simulink model "WiperControl"  (R2023b)
settings: Solver=FixedStepAuto  StartTime=0.0  StopTime=20  FixedStep=0.01  RelTol=1e-3
libraries: simulink x1, SignalEditorBlockLib x1
settings Model: LastModifiedBy=Mohamed Majdi
settings OptimizationCC: DefaultParameterBehavior=Inlined  UseDivisionForNetSlopeComputation=on  GainParamInheritBuiltInType=on  UseFloatMulNetSlope=on  OptimizeBlockIOStorage=off  LifeSpan=1  OptimizeDataStoreBuffers=off  BusAssignmentInplaceUpdate=off
settings DebuggingCC: SFUnexpectedBacktrackingDiag=warning  SFNoUnconditionalDefaultTransitionDiag=warning
settings HardwareCC: ProdLongLongMode=on
settings SFSimCC: MATLABDynamicMemAlloc=off
settings RTWCC: GenerateReport=on  BuildConfiguration=Debug  LaunchReport=on
settings CodeAppCC: ForceParamTrailComments=on  MATLABSourceComments=on  EnableCustomComments=on
settings GRTTargetCC: CombineSignalStateStructs=on  SupportVariableSizeSignals=on  MultiInstanceErrorCode=Warning

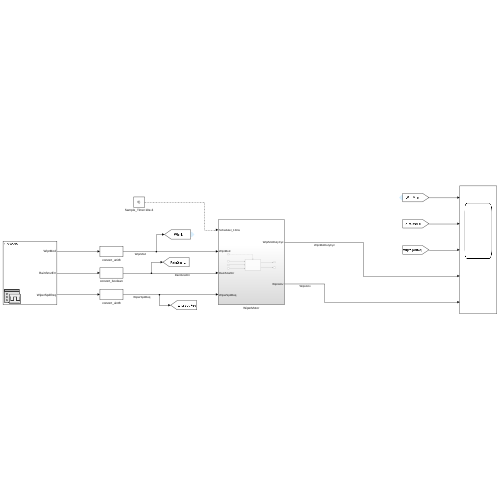
[thumbnail: Simulink's stored preview of the top-level diagram]
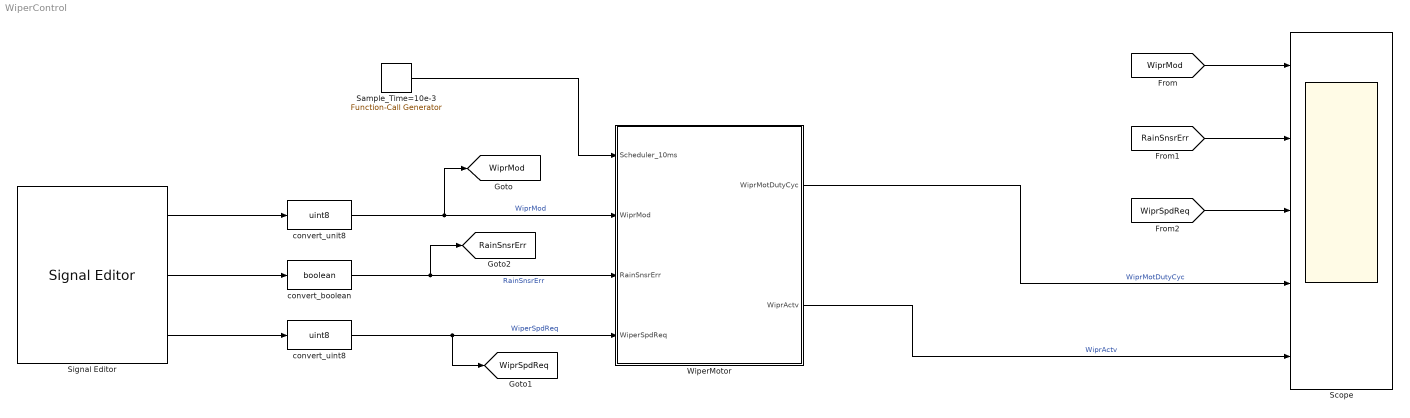
== system WiperControl ==
  Sample_Time=10e-3 : simulink/Ports & Subsystems/Function-Call Generator  sample_time=10e-3  numberOfIterations=1  DisallowWideOutput=off
  Scope : Scope  NumInputPorts=5
  Signal Editor : SignalEditorBlockLib/Signal Editor  FileName=WiperSignals.mat  ActiveScenario=Scenario  ActiveSignal=WiprMod  IsBus=off  OutputBusObjectStr=Bus: BusObject  SampleTime=0  Interpolate=off  ZeroCross=off  OutputAfterFinalValue=Setting to zero  Unit=inherit  PreserveSignalName=on  ApplySigPropsToAllScenarios=on  ApplySigPropsToAllSignals=on
  WiperMotor : Subsystem
  convert_boolean : DataTypeConversion  OutDataTypeStr=boolean  SaturateOnIntegerOverflow=off  RndMeth=Floor
  convert_uint8 : DataTypeConversion  OutDataTypeStr=uint8  SaturateOnIntegerOverflow=off  RndMeth=Floor
  convert_unit8 : DataTypeConversion  OutDataTypeStr=uint8  SaturateOnIntegerOverflow=off  RndMeth=Floor
  tag scope: RainSnsrErr=global, WiprMod=global, WiprSpdReq=global
  wires:
  convert_unit8/1 -> WiperMotor/2(WiprMod), [WiprMod]  "WiprMod"
  Signal Editor/3 -> convert_uint8/1
  Signal Editor/2 -> convert_boolean/1
  Signal Editor/1 -> convert_unit8/1
  [WiprMod] -> Scope/1
  Sample_Time=10e-3/1 -> WiperMotor/1(Scheduler_10ms)
  convert_boolean/1 -> [RainSnsrErr], WiperMotor/3(RainSnsrErr)  "RainSnsrErr"
  convert_uint8/1 -> WiperMotor/4(WiperSpdReq), [WiprSpdReq]  "WiperSpdReq"
  WiperMotor/1(WiprMotDutyCyc) -> Scope/4  "WiprMotDutyCyc"
  WiperMotor/2(WiprActv) -> Scope/5  "WiprActv"
  [RainSnsrErr] -> Scope/2
  [WiprSpdReq] -> Scope/3

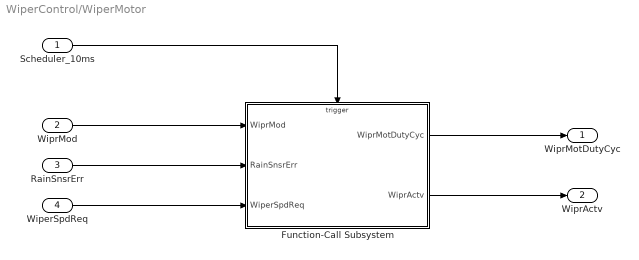
== system WiperControl/WiperMotor ==
  Scheduler_10ms : Inport
  WiprMod : Inport  Port=2  OutDataTypeStr=uint8
  RainSnsrErr : Inport  Port=3  OutDataTypeStr=boolean
  WiperSpdReq : Inport  Port=4  OutDataTypeStr=uint8
  Function-Call Subsystem : Subsystem  TreatAsAtomicUnit=on
  WiprMotDutyCyc : Outport
  WiprActv : Outport  Port=2  OutDataTypeStr=boolean
  wires:
  WiperSpdReq/1 -> Function-Call Subsystem/3(WiperSpdReq)
  Function-Call Subsystem/1(WiprMotDutyCyc) -> WiprMotDutyCyc/1
  Scheduler_10ms/1 -> Function-Call Subsystem/Trigger
  RainSnsrErr/1 -> Function-Call Subsystem/2(RainSnsrErr)
  WiprMod/1 -> Function-Call Subsystem/1(WiprMod)
  Function-Call Subsystem/2(WiprActv) -> WiprActv/1

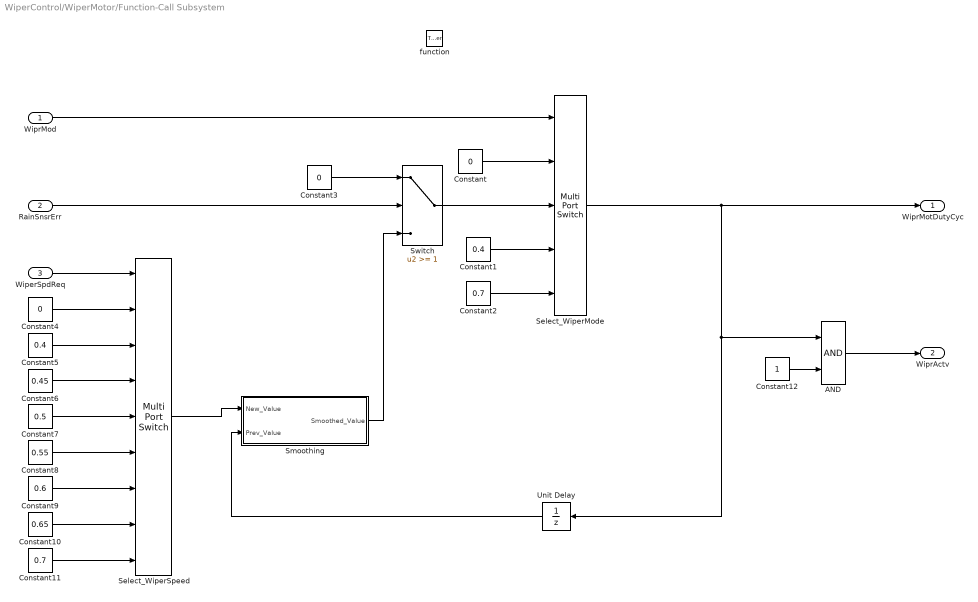
== system WiperControl/WiperMotor/Function-Call Subsystem ==
  WiprMod : Inport
  RainSnsrErr : Inport  Port=2
  WiperSpdReq : Inport  Port=3
  function : TriggerPort  TriggerType=function-call  VariantControl=(inherit)
  AND : Logic  IconShape=distinctive  AllPortsSameDT=off  OutDataTypeStr=boolean
  Constant : Constant  Value=0  OutDataTypeStr=uint8
  Constant1 : Constant  Value=0.4
  Constant10 : Constant  Value=0.65
  Constant11 : Constant  Value=0.7
  Constant12 : Constant
  Constant2 : Constant  Value=0.7
  Constant3 : Constant  Value=0  OutDataTypeStr=uint8
  Constant4 : Constant  Value=0
  Constant5 : Constant  Value=0.4
  Constant6 : Constant  Value=0.45
  Constant7 : Constant  Value=0.5
  Constant8 : Constant  Value=0.55
  Constant9 : Constant  Value=0.6
  Select_WiperMode : MultiPortSwitch  DataPortOrder=Zero-based contiguous  Inputs=4  zeroidx=on  SaturateOnIntegerOverflow=off  InputSameDT=off
  Select_WiperSpeed : MultiPortSwitch  DataPortOrder=Zero-based contiguous  Inputs=8  zeroidx=on  SaturateOnIntegerOverflow=off  InputSameDT=off
  Smoothing : Subsystem  TreatAsAtomicUnit=on
  Switch : Switch  Threshold=1  SaturateOnIntegerOverflow=off  InputSameDT=off
  Unit Delay : UnitDelay  SampleTime=-1  HasFrameUpgradeWarning=on
  WiprMotDutyCyc : Outport  OutDataTypeStr=double
  WiprActv : Outport  Port=2  OutDataTypeStr=boolean
  wires:
  WiprMod/1 -> Select_WiperMode/1
  Select_WiperMode/1 -> WiprMotDutyCyc/1, Unit Delay/1, AND/1
  Constant/1 -> Select_WiperMode/2
  Constant2/1 -> Select_WiperMode/5
  Constant1/1 -> Select_WiperMode/4
  RainSnsrErr/1 -> Switch/2
  Switch/1 -> Select_WiperMode/3
  Constant3/1 -> Switch/1
  WiperSpdReq/1 -> Select_WiperSpeed/1
  Constant4/1 -> Select_WiperSpeed/2
  Constant5/1 -> Select_WiperSpeed/3
  Constant6/1 -> Select_WiperSpeed/4
  Constant7/1 -> Select_WiperSpeed/5
  Constant8/1 -> Select_WiperSpeed/6
  Constant9/1 -> Select_WiperSpeed/7
  Constant10/1 -> Select_WiperSpeed/8
  Constant11/1 -> Select_WiperSpeed/9
  AND/1 -> WiprActv/1
  Constant12/1 -> AND/2
  Select_WiperSpeed/1 -> Smoothing/1(New_Value)
  Unit Delay/1 -> Smoothing/2(Prev_Value)
  Smoothing/1(Smoothed_Value) -> Switch/3

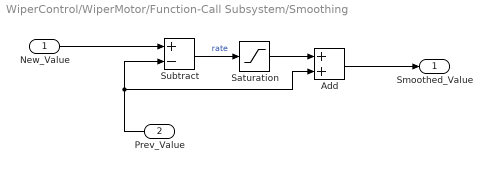
== system WiperControl/WiperMotor/Function-Call Subsystem/Smoothing ==
  New_Value : Inport
  Prev_Value : Inport  Port=2
  Add : Sum
  Saturation : Saturate  UpperLimit=0.005  LowerLimit=-0.005
  Subtract : Sum  Inputs=+-
  Smoothed_Value : Outport
  wires:
  Saturation/1 -> Add/1
  Prev_Value/1 -> Subtract/2, Add/2
  New_Value/1 -> Subtract/1
  Subtract/1 -> Saturation/1  "rate"
  Add/1 -> Smoothed_Value/1
